simulink model "Tut01"  (R2024a)
settings: Solver=VariableStepAuto  StartTime=0.0  StopTime=10.0  FixedStep=6  RelTol=1e-3
settings Model: Creator=User  LastModifiedBy=User
settings OptimizationCC: DefaultParameterBehavior=Inlined  UseDivisionForNetSlopeComputation=on  GainParamInheritBuiltInType=on  UseFloatMulNetSlope=on  InlineInvariantSignals=on  PassReuseOutputArgsAs=Individual arguments  ZeroExternalMemoryAtStartup=off  ZeroInternalMemoryAtStartup=off  NoFixptDivByZeroProtection=on  EfficientFloat2IntCast=on  LifeSpan=1  OptimizeBlockOrder=speed  DifferentSizesBufferReuse=on  EfficientTunableParamExpr=on
settings DebuggingCC: ParameterTunabilityLossMsg=error
settings HardwareCC: ProdBitPerInt=16  ProdBitPerPointer=16  ProdBitPerSizeT=16  ProdBitPerPtrDiffT=16  ProdLargestAtomicFloat=None  ProdWordSize=16  ProdLongLongMode=on  ProdHWDeviceType=Atmel->AVR (8-bit)
settings SFSimCC: MATLABDynamicMemAlloc=off
settings RTWCC: Description=Embedded Coder  SystemTargetFile=ert.tlc  TemplateMakefile=ert_default_tmf
settings CodeAppCC: ForceParamTrailComments=on  IgnoreCustomStorageClasses=off  OperatorAnnotations=on  SimulinkDataObjDesc=on  SFDataObjDesc=on  CustomSymbolStrGlobalVar=rt$N$M  CustomSymbolStrType=$N$M  CustomSymbolStrFcn=$N$M$F  CustomSymbolStrMacro=$N$M  InsertBlockDesc=on
settings ERTTargetCC: TargetLangStandard=C99 (ISO)  GenerateSampleERTMain=on  IncludeMdlTerminateFcn=off  CombineSignalStateStructs=on  SupportComplex=off  SupportContinuousTime=on  SupportNonInlinedSFcns=on  InlinedParameterPlacement=NonHierarchical  ERTCustomFileTemplate=example_file_process.tlc  ERTFilePackagingFormat=CompactWithDataFile

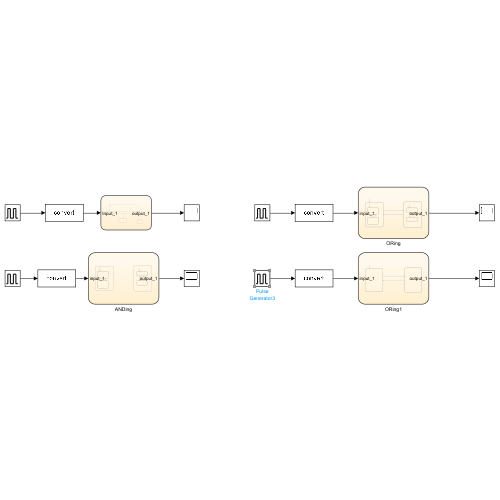
[thumbnail: Simulink's stored preview of the top-level diagram]
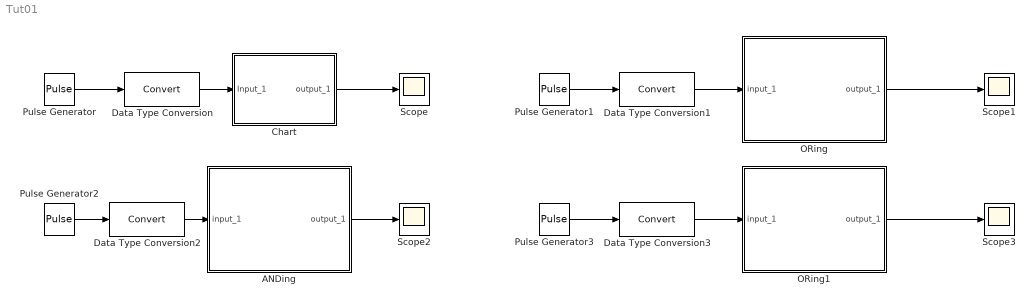
== system Tut01 ==
  ANDing : Stateflow chart  TreatAsAtomicUnit=on
  Chart : Stateflow chart  TreatAsAtomicUnit=on
  Data Type Conversion{,1..3} (4 alike) : DataTypeConversion  SaturateOnIntegerOverflow=off  RndMeth=Floor
  ORing : Stateflow chart  TreatAsAtomicUnit=on
  ORing1 : Stateflow chart  TreatAsAtomicUnit=on
  Pulse Generator{,1..3} (4 alike) : DiscretePulseGenerator  PulseType=Time based  PulseWidth=50
  Scope{,1..3} (4 alike) : Scope
  wires:
  Chart/1(output_1) -> Scope/1
  Pulse Generator/1 -> Data Type Conversion/1
  Data Type Conversion/1 -> Chart/1(Input_1)
  Pulse Generator1/1 -> Data Type Conversion1/1
  Data Type Conversion1/1 -> ORing/1(input_1)
  ORing/1(output_1) -> Scope1/1
  ANDing/1(output_1) -> Scope2/1
  Data Type Conversion2/1 -> ANDing/1(input_1)
  Pulse Generator2/1 -> Data Type Conversion2/1
  ORing1/1(output_1) -> Scope3/1
  Data Type Conversion3/1 -> ORing1/1(input_1)
  Pulse Generator3/1 -> Data Type Conversion3/1

== stateflow chart Tut01/ORing ==
  state OFF_State
    state OFF_1
    state OFF_2
    (default) -> OFF_1
    OFF_1 -> OFF_2
    OFF_2 -> OFF_1
  state ON_State
    state ON_1
    state ON_2
    (default) -> ON_1
    ON_1 -> ON_2
    ON_2 -> ON_1
  (default) -> ON_State
  ON_State -> OFF_State : [input_1 == 1]
  OFF_State -> ON_State : [input_1 == 0]
  data: input_1 input uint8 size=[1 1]; output_1 output boolean size=[1 1]

== stateflow chart Tut01/ANDing ==
  state OFF_State [parallel]
    settings: executionOrder=1
    state OFF_1
    state OFF_2
    (default) -> OFF_1
    OFF_1 -> OFF_2
    OFF_2 -> OFF_1
  state ON_State [parallel]
    settings: executionOrder=2
    state ON_1
    state ON_2
    (default) -> ON_1
    ON_1 -> ON_2
    ON_2 -> ON_1
  data: input_1 input uint8 size=[1 1]; output_1 output boolean size=[1 1]

== stateflow chart Tut01/Chart ==
  state IN
    output_1=1;
    local_1=parameter_1;
  state OUT
    output_1=0;
  state ON2
  state OUT1
    output_1=0;
  (default) -> (junction 18)
  (junction 18) -> OUT [order 1] : [Input_1 == 4]
  (junction 18) -> IN [order 2]
  IN -> OUT : after(3,tick) [hasChanged(Input_1)]{local_1 = 2;}/{output_1=1;}
  (junction 21) -> IN [order 1] : [hasChanged(Input_1)]
  OUT -> (junction 21) [order 1] : [ Input_1 == 1 ]
  (junction 21) -> ON2 [order 2]
  OUT1 -> OUT : after(3,tick)
  OUT -> OUT1 [order 2] : after(4,tick)
  data: Input_1 input uint8; local_1 local double size=[1 1] =0; parameter_1 parameter double; output_1 output double; data_const constant double size=[1 1]

== stateflow chart Tut01/ORing1 ==
  state OFF_State
    en:
    local_1=2;
    du:
    output_1=1;
    ex:
    output_1=4;
  state ON_State
    en:
    local_1=4;
    du:
    output_1=3;
    ex:
    output_1=2;
  (default) -> ON_State
  ON_State -> OFF_State : [input_1 == 1]
  OFF_State -> ON_State : [input_1 == 0]
  data: input_1 input uint8 size=[1 1]; output_1 output boolean size=[1 1]; local_1 local uint8
